simulink model "arm_sim_loop"  (Simulink 7.7)
settings: Solver=ode45  StartTime=0.0  StopTime=100  RelTol=1e-3
undefined symbols (not defined in the file or in its folder): arm_ctrl_loop, drawArm, P
libraries: simulink x1
settings Model: Creator=beard  LastModifiedBy=beard
settings OptimizationCC: InitFltsAndDblsToZero=on
settings DebuggingCC: StrictBusMsg=Warning

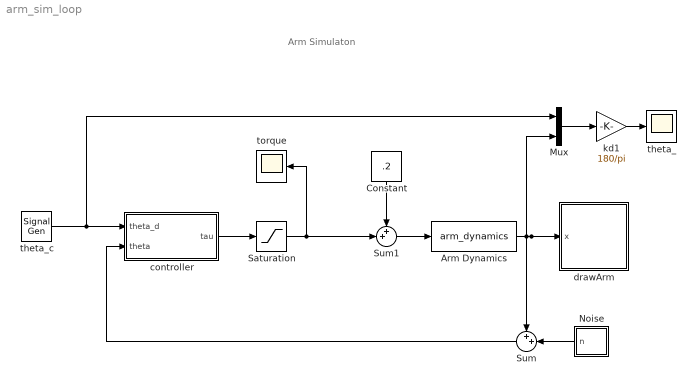
== system arm_sim_loop ==
  note: Arm Simulaton
  Arm Dynamics : S-Function  FunctionName=arm_dynamics  Parameters=AP  EnableBusSupport=off
  Constant : Constant  Value=.2
  Mux : Mux  Inputs=2
  Noise : Subsystem
  Saturation : Saturate  UpperLimit=P.tau_max  LowerLimit=-P.tau_max
  Sum : Sum  Inputs=++|
  Sum1 : Sum  Inputs=++|
  controller : Subsystem
  drawArm : Subsystem
      mask init:
      | % drawing parameters
      | L = 1;
      | w = 0.3;
      mask Display: image(imread('tv.jpg'))
  kd1 : Gain  Gain=180/pi
  theta_ : Scope
      settings: YMin=-40  YMax=50
  theta_c : SignalGenerator  WaveForm=square  Amplitude=25*pi/180  Frequency=.05
  torque : Scope
      settings: YMin=-0.1  YMax=1
  wires:
  Arm Dynamics/1 -> drawArm/1(x), Sum/1, Mux/2
  Mux/1 -> kd1/1
  kd1/1 -> theta_/1
  controller/1(tau) -> Saturation/1
  theta_c/1 -> controller/1(theta_d), Mux/1
  Sum/1 -> controller/2(theta)
  Saturation/1 -> Sum1/2, torque/1
  Sum1/1 -> Arm Dynamics/1
  Noise/1(n) -> Sum/2
  Constant/1 -> Sum1/1

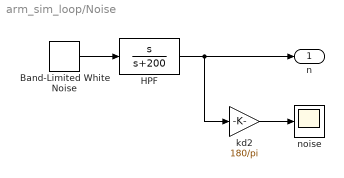
== system arm_sim_loop/Noise ==
  Band-Limited White Noise : simulink/Sources/Band-Limited White Noise  SystemSampleTime=-1  Cov=[0.000001]  Ts=P.Ts  seed=[23341]
  HPF : TransferFcn  Numerator=[1 0]  Denominator=[1 200]
  kd2 : Gain  Gain=180/pi
  noise : Scope
      settings: YMin=-7  YMax=8  SaveName=ScopeData2
  n : Outport
  wires:
  Band-Limited White Noise/1 -> HPF/1
  kd2/1 -> noise/1
  HPF/1 -> kd2/1, n/1

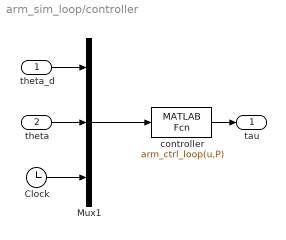
== system arm_sim_loop/controller ==
  theta_d : Inport
  theta : Inport  Port=2
  Clock : Clock
      settings: Decimation=10
  Mux1 : Mux  Inputs=3
  controller : MATLABFcn  MATLABFcn=arm_ctrl_loop(u,P)  OutputDimensions=1  SampleTime=P.Ts
  tau : Outport
  wires:
  Mux1/1 -> controller/1
  theta_d/1 -> Mux1/1
  theta/1 -> Mux1/2
  controller/1 -> tau/1
  Clock/1 -> Mux1/3

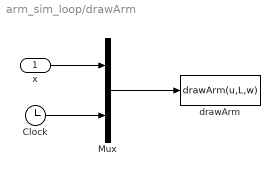
== system arm_sim_loop/drawArm ==
  x : Inport
  Clock : Clock
      settings: Decimation=10
  Mux : Mux  Inputs=2
  drawArm : MATLABFcn  MATLABFcn=drawArm(u,L,w)  OutputDimensions=0  SampleTime=0.1
  wires:
  Mux/1 -> drawArm/1
  x/1 -> Mux/1
  Clock/1 -> Mux/2
